simulink model "VirtualVehicleTemplate"  (R2024a)
settings: configuration reference "VehicleVariable" (kept outside this file)
StartFcn:
  | %tic
StopFcn:
  | %toc
model workspace (MAT data in the model file):
  ExtDrvCmdsSwitch : Simulink.Parameter (value not decoded)
  ExtDrvRefSwitch : Simulink.Parameter (value not decoded)
  ExtEnvSwitch : Simulink.Parameter (value not decoded)
  ExtGndSwitch : Simulink.Parameter (value not decoded)
symbols that are objects in the model workspace (value not decoded): ExtDrvCmdsSwitch, ExtDrvRefSwitch, ExtEnvSwitch, ExtGndSwitch
undefined symbols (not defined in the file): AccelCmd, AmbTemp, BaroPress, CurvGradRef, CurvRef, DCM, DecelCmd, Disabled, DriverAeroRes, DriverDrivelineRes, DriverInitialGear, DriverPreviewDist, DriverRollRes, DriverShiftTime, DriverTimeConst, DriverTractiveForce, EnvAbsPrs, EnvAirTemp, EnvGrvty, EnvNomFrictionScaling, EnvNominalGrade, EnvWindVelX, EnvWindVelY, EnvWindVelZ, FTP75, Gnd, Grade, HazzardCmd, HighBeamCmd, lambda_mux, LeftSignalCmd, LngRef, LowBeamCmd, LtrRef, PhiRef, PlntVehDstCGFrntAxl, PlntVehDstCGRearAxl, PlntVehInitLatPos, PlntVehInitLongPos, PlntVehInitPitchAng, PlntVehInitRollAng, PlntVehInitVertPos, PlntVehInitYawAng, PlntVehMass, PlntVehTrckWdth, PlntVehYawMomentInertia, PlntWhlLdRadius, RightSignalCmd, ScnCRMaxLatAccel, ScnCRRadius, ScnDLCGateLongPos, ScnDLCLatRef, ScnDLCLatRefOffset, ScnDLCLongRefBpt, ScnDLCLongRefStartPos, ScnDLCVehicleWidth, ScnFHCounterDwellTime, ScnFHInitialDwellTime, ScnFHReturnTime, ScnFHRollRateZeroCross ... (+20)
libraries: simulink x27, autolibutils x8, vehdynlibscenariocommon x7, vehdynlibviscommon x4, autolibshared x3, vehdynlibdriver x2, sim3dgroundtruthsensorlib x2, sim3dautolib x2, vrlib x1, autolibsharedcommon x1, sharedtransform x1, sim3dlib x1
(part 2 of 6)

== system VirtualVehicleTemplate/Controllers/TCU Input ==
  CntrlRx : Inport
  Brake : Inport  Port=2
  Bus Selector : BusSelector  OutputSignals=ABSFlag
  Bus Selector1 : BusSelector  OutputSignals=Driver.AccelFdbk,Driver.DecelFdbk,Driver.GearFdbk,Trans.Info.Eng.EngSpd,FrntWheels.Wheels.Omega,RearWheels.Wheels.Omega,Body.BdyFrm.Cg.Vel.xdot
  Bus to Vector : BusToVector
  Bus to Vector1 : BusToVector
  Ground : Ground
  Ground1 : Ground
  Rate Transition{1..8,23} (9 alike) : RateTransition  Deterministic=off
  Vector Concatenate : Concatenate
  <AccFdbk> : Outport
  <DecelFdbk> : Outport  Port=2
  <GearFdbk> : Outport  Port=3
  <EngSpd> : Outport  Port=4
  <Omega> : Outport  Port=5
  <Vehicle> : Outport  Port=6
  ABSFlag : Outport  Port=7
  UpReq : Outport  Port=8
  DnReq : Outport  Port=9
  wires:
  Bus Selector1/7 -> Rate Transition5/1  "<xdot>"
  Bus Selector1/2 -> Rate Transition1/1  "<DecelFdbk>"
  Ground/1 -> Rate Transition7/1
  CntrlRx/1 -> Bus Selector1/1
  Bus Selector1/1 -> Rate Transition23/1  "<AccelFdbk>"
  Vector Concatenate/1 -> Rate Transition4/1
  Bus Selector1/4 -> Rate Transition3/1  "<EngSpd>"
  Bus Selector1/3 -> Rate Transition2/1  "<GearFdbk>"
  Ground1/1 -> Rate Transition8/1
  Bus Selector/1 -> Rate Transition6/1  "<ABSFlag>"
  Brake/1 -> Bus Selector/1
  Rate Transition23/1 -> <AccFdbk>/1
  Rate Transition1/1 -> <DecelFdbk>/1
  Rate Transition2/1 -> <GearFdbk>/1
  Rate Transition3/1 -> <EngSpd>/1
  Rate Transition4/1 -> <Omega>/1
  Rate Transition5/1 -> <Vehicle>/1
  Rate Transition6/1 -> ABSFlag/1
  Rate Transition7/1 -> UpReq/1
  Rate Transition8/1 -> DnReq/1
  Bus Selector1/5 -> Bus to Vector/1  "<Omega>"
  Bus Selector1/6 -> Bus to Vector1/1  "<Omega>"
  Bus to Vector/1 -> Vector Concatenate/1
  Bus to Vector1/1 -> Vector Concatenate/2

== system VirtualVehicleTemplate/Controllers/TCU Output ==
  GearCmd : Inport
  Bus Creator1 : BusCreator  Inputs=1
  First Order Hold : FirstOrderHold  ErrorTolerance=inf
  Trans : Outport
  wires:
  Bus Creator1/1 -> Trans/1  "Trans"
  GearCmd/1 -> First Order Hold/1  "GearCmd"
  First Order Hold/1 -> Bus Creator1/1  "GearCmd"

== system VirtualVehicleTemplate/Controllers/Thermal Input ==
  Bus Element In : Inport  PortName=CntrlRx  Element=Thermal.BattCoolTemp
  Bus Element In2 : Inport  PortName=CntrlRx  Element=Thermal.CondPress
  Bus Element In3 : Inport  PortName=CntrlRx  Element=Thermal.ChlrPress
  Bus Element In5 : Inport  PortName=CntrlRx  Element=Thermal.MotorTemp
  Bus Element In6 : Inport  PortName=CntrlRx  Element=Thermal.BattTemp
  Bus Element In7 : Inport  PortName=CntrlRx  Element=Thermal.InvCoolTempOut
  Bus Element In8 : Inport  PortName=CntrlRx  Element=Thermal.InvTemp
  Bus Element In1 : Inport  PortName=CntrlRx  Element=Battery.BMSSensors.CellTemperatures
  Bus Element In4 : Inport  PortName=CntrlRx  Element=Env.AmbTemp
  Rate Transition{,1..8} (9 alike) : RateTransition
  CoolTemp : Outport
  CellTemps : Outport  Port=2
  AmbTemp : Outport  Port=3
  CondPress : Outport  Port=4
  ChlrPress : Outport  Port=5
  MotorTemp : Outport  Port=6
  BattTemp : Outport  Port=7
  InvCoolTempOut : Outport  Port=8
  InvTemp : Outport  Port=9
  wires:
  Bus Element In/1 -> Rate Transition/1
  Bus Element In1/1 -> Rate Transition8/1
  Rate Transition/1 -> CoolTemp/1
  Bus Element In2/1 -> Rate Transition1/1
  Rate Transition1/1 -> CondPress/1
  Rate Transition2/1 -> ChlrPress/1
  Bus Element In3/1 -> Rate Transition2/1
  Rate Transition3/1 -> AmbTemp/1
  Bus Element In4/1 -> Rate Transition3/1
  Rate Transition4/1 -> MotorTemp/1
  Bus Element In5/1 -> Rate Transition4/1
  Rate Transition5/1 -> BattTemp/1
  Bus Element In6/1 -> Rate Transition5/1
  Rate Transition6/1 -> InvCoolTempOut/1
  Bus Element In7/1 -> Rate Transition6/1
  Rate Transition7/1 -> InvTemp/1
  Bus Element In8/1 -> Rate Transition7/1
  Rate Transition8/1 -> CellTemps/1

== system VirtualVehicleTemplate/Controllers/Thermal Management ==
  CoolTemp : Inport
  CellTemps : Inport  Port=2
  AmbTemp : Inport  Port=3  Unit=K
  CondPress : Inport  Port=4
  ChlrPress : Inport  Port=5
  MotorTemp : Inport  Port=6
  BattTemp : Inport  Port=7
  InvCoolTempOut : Inport  Port=8
  InvTemp : Inport  Port=9
  NoThermalControl : ModelReference  ModelNameDialog=NoThermalControl  SimulationMode=Normal  VariantControl=NoThermalControl  ModelReferenceVersion=2.28
  ThermalControl : ModelReference  ModelNameDialog=ThermalControl.slx  SimulationMode=Normal  VariantControl=ThermalControl  ModelReferenceVersion=2.119
  ThermalControlGen1 : ModelReference  ModelNameDialog=ThermalControlGen1  SimulationMode=Normal  VariantControl=ThermalControlGen1  ModelReferenceVersion=2.30
  ValveCmd : Outport
  PumpCmd : Outport  Port=2
  CmpCmd : Outport  Port=3
  FanCmd : Outport  Port=4
  HeaterCmd : Outport  Port=5
  MotPmpCmd : Outport  Port=6
  BattPmpCmd : Outport  Port=7
  ChlrByPCmd : Outport  Port=8
  SerParCmd : Outport  Port=9
  RadByPCmd : Outport  Port=10

== system VirtualVehicleTemplate/Controllers/Thermal Output ==
  ValveCmd : Inport
  PumpCmd : Inport  Port=2
  CmpCmd : Inport  Port=3
  FanCmd : Inport  Port=4
  HeaterCmd : Inport  Port=5
  MotPmpCmd : Inport  Port=6
  BattPmpCmd : Inport  Port=7
  ChlrPyPCmd : Inport  Port=8
  SerParCmd : Inport  Port=9
  RadByPCmd : Inport  Port=10
  First Order Hold{,1..9} (10 alike) : FirstOrderHold  ErrorTolerance=inf
  Bus Element Out : Outport  PortName=Thermal  Element=ValveCmd
  Bus Element Out1 : Outport  PortName=Thermal  Element=PumpCmd
  Bus Element Out2 : Outport  PortName=Thermal  Element=CmpCmd
  Bus Element Out3 : Outport  PortName=Thermal  Element=FanCmd
  Bus Element Out4 : Outport  PortName=Thermal  Element=HeaterCmd
  Bus Element Out5 : Outport  PortName=Thermal  Element=MotPmpCmd
  Bus Element Out6 : Outport  PortName=Thermal  Element=BattPmpCmd
  Bus Element Out7 : Outport  PortName=Thermal  Element=ChlrByPCmd
  Bus Element Out8 : Outport  PortName=Thermal  Element=SerParCmd
  Bus Element Out9 : Outport  PortName=Thermal  Element=RadByPCmd
  wires:
  PumpCmd/1 -> First Order Hold1/1
  ValveCmd/1 -> First Order Hold/1
  First Order Hold/1 -> Bus Element Out/1
  First Order Hold1/1 -> Bus Element Out1/1
  CmpCmd/1 -> First Order Hold2/1
  First Order Hold2/1 -> Bus Element Out2/1
  First Order Hold3/1 -> Bus Element Out3/1
  FanCmd/1 -> First Order Hold3/1
  HeaterCmd/1 -> First Order Hold4/1
  First Order Hold4/1 -> Bus Element Out4/1
  MotPmpCmd/1 -> First Order Hold5/1
  First Order Hold5/1 -> Bus Element Out5/1
  BattPmpCmd/1 -> First Order Hold6/1
  First Order Hold6/1 -> Bus Element Out6/1
  ChlrPyPCmd/1 -> First Order Hold7/1
  First Order Hold7/1 -> Bus Element Out7/1
  First Order Hold8/1 -> Bus Element Out8/1
  SerParCmd/1 -> First Order Hold8/1
  First Order Hold9/1 -> Bus Element Out9/1
  RadByPCmd/1 -> First Order Hold9/1

== system VirtualVehicleTemplate/Controllers/Transmission Control Unit (TCU) ==
  Accel : Inport
  BrkCmd : Inport  Port=2
  GearReq : Inport  Port=3
  EngSpd : Inport  Port=4
  Omega : Inport  Port=5  Unit=rad/s
  VehSpdFdbk : Inport  Port=6
  ABSFlag : Inport  Port=7
  UpReq : Inport  Port=8
  DownReq : Inport  Port=9  Unit=rad/s
  DriverPassThrough : ModelReference  ModelNameDialog=DriverPassThrough.slx  VariantControl=DriverPassThrough  ModelReferenceVersion=8.0
  TransmissionController : ModelReference  ModelNameDialog=TransmissionController  VariantControl=TransmissionController  ModelReferenceVersion=8.8
  " Gear" : Outport  VectorParamsAs1DForOutWhenUnconnected=off

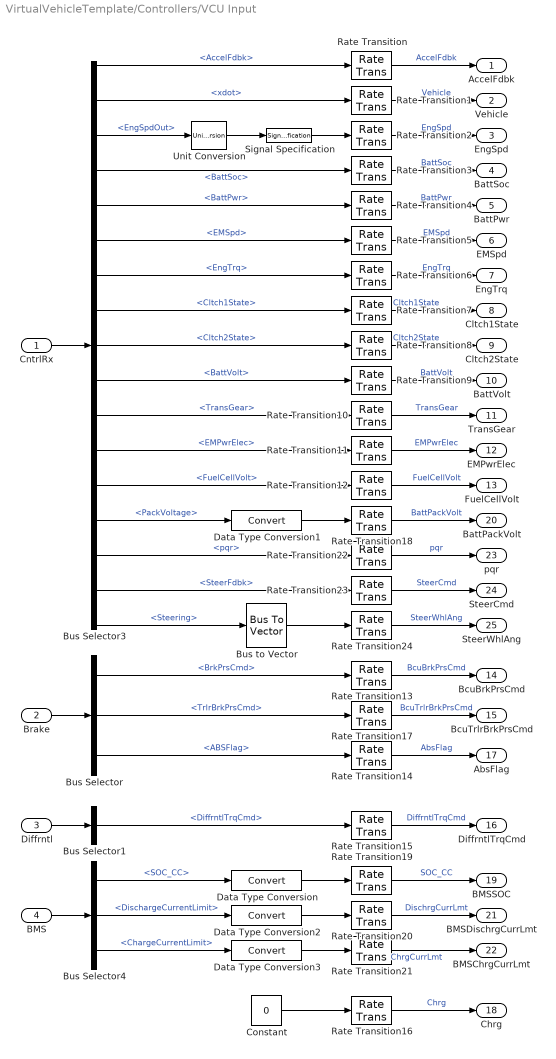
== system VirtualVehicleTemplate/Controllers/VCU Input ==
  CntrlRx : Inport
  Brake : Inport  Port=2
  Diffrntl : Inport  Port=3
  BMS : Inport  Port=4
  Bus Selector : BusSelector  OutputSignals=BrkPrsCmd,TrlrBrkPrsCmd,ABSFlag
  Bus Selector1 : BusSelector  OutputSignals=DiffrntlTrqCmd
  Bus Selector3 : BusSelector  OutputSignals=Driver.AccelFdbk,Body.BdyFrm.Cg.Vel.xdot,Engine.EngSpdOut,Battery.BattInfo.BattSoc,Battery.BattInfo.BattPwr,EM.EMSpd,Engine.EngTrq,Trans.Cltch1State,Trans.Cltch2State,Battery.BattInfo.BattVolt,Trans.Info.Trans.TransGear,EM.EMPwrElec,FuelCell.FuelCellVolt,Battery.BMSSensors.PackVoltage,IMU.pqr,Driver.SteerFdbk,Steering
  Bus Selector4 : BusSelector  OutputSignals=BMSInfo.SOC.SOC_CC,BMSCmd.CurrentLimitsBus.DischargeCurrentLimit,BMSCmd.CurrentLimitsBus.ChargeCurrentLimit
  Bus to Vector : BusToVector
  Constant : Constant  Value=0  SampleTime=-1
  Data Type Conversion{,1..3} (4 alike) : DataTypeConversion  SaturateOnIntegerOverflow=off  RndMeth=Floor
  Rate Transition{,1..24} (25 alike) : RateTransition  Deterministic=off
  Signal Specification : SignalSpecification  Unit=rad/s
  Unit Conversion : UnitConversion
  AccelFdbk : Outport
  Vehicle : Outport  Port=2
  EngSpd : Outport  Port=3
  BattSoc : Outport  Port=4
  BattPwr : Outport  Port=5
  EMSpd : Outport  Port=6
  EngTrq : Outport  Port=7
  Cltch1State : Outport  Port=8
  Cltch2State : Outport  Port=9
  BattVolt : Outport  Port=10
  TransGear : Outport  Port=11
  EMPwrElec : Outport  Port=12
  FuelCellVolt : Outport  Port=13
  BcuBrkPrsCmd : Outport  Port=14
  BcuTrlrBrkPrsCmd : Outport  Port=15
  DiffrntlTrqCmd : Outport  Port=16
  AbsFlag : Outport  Port=17
  Chrg : Outport  Port=18
  BMSSOC : Outport  Port=19
  BattPackVolt : Outport  Port=20
  BMSDischrgCurrLmt : Outport  Port=21
  BMSChrgCurrLmt : Outport  Port=22
  pqr : Outport  Port=23
  SteerCmd : Outport  Port=24
  SteerWhlAng : Outport  Port=25
  wires:
  Bus Selector3/5 -> Rate Transition4/1  "<BattPwr>"
  Bus Selector3/1 -> Rate Transition/1  "<AccelFdbk>"
  Bus Selector3/7 -> Rate Transition6/1  "<EngTrq>"
  Bus Selector3/4 -> Rate Transition3/1  "<BattSoc>"
  Bus Selector3/6 -> Rate Transition5/1  "<EMSpd>"
  CntrlRx/1 -> Bus Selector3/1
  Bus Selector3/11 -> Rate Transition10/1  "<TransGear>"
  Bus Selector3/9 -> Rate Transition8/1  "<Cltch2State>"
  Bus Selector3/13 -> Rate Transition12/1  "<FuelCellVolt>"
  Bus Selector3/2 -> Rate Transition1/1  "<xdot>"
  Bus Selector3/8 -> Rate Transition7/1  "<Cltch1State>"
  Bus Selector3/10 -> Rate Transition9/1  "<BattVolt>"
  Bus Selector3/3 -> Unit Conversion/1  "<EngSpdOut>"
  Bus Selector3/12 -> Rate Transition11/1  "<EMPwrElec>"
  Bus Selector/1 -> Rate Transition13/1  "<BrkPrsCmd>"
  Constant/1 -> Rate Transition16/1
  Brake/1 -> Bus Selector/1
  Bus Selector/3 -> Rate Transition14/1  "<ABSFlag>"
  Diffrntl/1 -> Bus Selector1/1
  Bus Selector1/1 -> Rate Transition15/1  "<DiffrntlTrqCmd>"
  Rate Transition/1 -> AccelFdbk/1  "AccelFdbk"
  Rate Transition1/1 -> Vehicle/1  "Vehicle"
  Rate Transition2/1 -> EngSpd/1  "EngSpd"
  Rate Transition3/1 -> BattSoc/1  "BattSoc"
  Rate Transition4/1 -> BattPwr/1  "BattPwr"
  Rate Transition5/1 -> EMSpd/1  "EMSpd"
  Rate Transition6/1 -> EngTrq/1  "EngTrq"
  Rate Transition7/1 -> Cltch1State/1  "Cltch1State"
  Rate Transition8/1 -> Cltch2State/1  "Cltch2State"
  Rate Transition9/1 -> BattVolt/1  "BattVolt"
  Rate Transition10/1 -> TransGear/1  "TransGear"
  Rate Transition11/1 -> EMPwrElec/1  "EMPwrElec"
  Rate Transition12/1 -> FuelCellVolt/1  "FuelCellVolt"
  Rate Transition13/1 -> BcuBrkPrsCmd/1  "BcuBrkPrsCmd"
  Rate Transition14/1 -> AbsFlag/1  "AbsFlag"
  Rate Transition15/1 -> DiffrntlTrqCmd/1  "DiffrntlTrqCmd"
  Rate Transition16/1 -> Chrg/1  "Chrg"
  Rate Transition20/1 -> BMSDischrgCurrLmt/1  "DischrgCurrLmt"
  Rate Transition19/1 -> BMSSOC/1  "SOC_CC"
  Rate Transition21/1 -> BMSChrgCurrLmt/1  "ChrgCurrLmt"
  Data Type Conversion3/1 -> Rate Transition21/1
  Data Type Conversion2/1 -> Rate Transition20/1
  Bus Selector4/1 -> Data Type Conversion/1  "<SOC_CC>"
  Data Type Conversion/1 -> Rate Transition19/1
  Bus Selector4/3 -> Data Type Conversion3/1  "<ChargeCurrentLimit>"
  Bus Selector4/2 -> Data Type Conversion2/1  "<DischargeCurrentLimit>"
  BMS/1 -> Bus Selector4/1
  Data Type Conversion1/1 -> Rate Transition18/1
  Rate Transition18/1 -> BattPackVolt/1  "BattPackVolt"
  Bus Selector3/14 -> Data Type Conversion1/1  "<PackVoltage>"
  Bus Selector/2 -> Rate Transition17/1  "<TrlrBrkPrsCmd>"
  Rate Transition17/1 -> BcuTrlrBrkPrsCmd/1  "BcuTrlrBrkPrsCmd"
  Rate Transition22/1 -> pqr/1  "pqr"
  Rate Transition23/1 -> SteerCmd/1  "SteerCmd"
  Rate Transition24/1 -> SteerWhlAng/1  "SteerWhlAng"
  Bus Selector3/15 -> Rate Transition22/1  "<pqr>"
  Bus Selector3/16 -> Rate Transition23/1  "<SteerFdbk>"
  Bus Selector3/17 -> Bus to Vector/1  "<Steering>"
  Unit Conversion/1 -> Signal Specification/1
  Signal Specification/1 -> Rate Transition2/1
  Bus to Vector/1 -> Rate Transition24/1

== system VirtualVehicleTemplate/Controllers/VCU Output ==
  EngTrqCmd : Inport
  EMTrqCmd : Inport  Port=2
  VcuBrkPrsCmd : Inport  Port=3
  VcuTrlrBrkPrsCmd : Inport  Port=4
  Cltch1Cmd : Inport  Port=5
  Neutral : Inport  Port=6
  FuelCellCurrCmd : Inport  Port=7
  FuelCellTempCmd : Inport  Port=8
  First Order Hold{,1..2,4..7} (7 alike) : FirstOrderHold  ErrorTolerance=inf
  First Order Hold3 : FirstOrderHold  ErrorTolerance=inf  AllowContinuousInput=on
  Out Bus Element : Outport  PortName=Vcu  Element=EngTrqCmd
  Out Bus Element1 : Outport  PortName=Vcu  Element=EMTrqCmd
  Out Bus Element2 : Outport  PortName=Vcu  Element=VcuBrkPrsCmd
  Out Bus Element3 : Outport  PortName=Vcu  Element=VcuTrlrBrkPrsCmd
  Out Bus Element4 : Outport  PortName=Vcu  Element=Cltch1Cmd
  Out Bus Element5 : Outport  PortName=Vcu  Element=Neutral
  Out Bus Element6 : Outport  PortName=Vcu  Element=FuelCellCurrCmd
  Out Bus Element7 : Outport  PortName=Vcu  Element=FuelCellTempCmd
  Out Bus Element8 : Outport  Port=2  PortName=VcuFdbk  Element=EngTrqCmd
  Out Bus Element9 : Outport  Port=2  PortName=VcuFdbk  Element=EMTrqCmd
  Out Bus Element10 : Outport  Port=2  PortName=VcuFdbk  Element=VcuBrkPrsCmd
  Out Bus Element11 : Outport  Port=2  PortName=VcuFdbk  Element=VcuTrlrBrkPrsCmd
  Out Bus Element12 : Outport  Port=2  PortName=VcuFdbk  Element=Cltch1Cmd
  Out Bus Element13 : Outport  Port=2  PortName=VcuFdbk  Element=Neutral
  Out Bus Element14 : Outport  Port=2  PortName=VcuFdbk  Element=FuelCellCurrCmd
  Out Bus Element15 : Outport  Port=2  PortName=VcuFdbk  Element=FuelCellTempCmd
  wires:
  Cltch1Cmd/1 -> Out Bus Element12/1, First Order Hold4/1  "Cltch1Cmd"
  EngTrqCmd/1 -> Out Bus Element8/1, First Order Hold/1  "EngTrqCmd"
  VcuBrkPrsCmd/1 -> Out Bus Element10/1, First Order Hold2/1  "VcuBrkPrsCmd"
  Neutral/1 -> Out Bus Element13/1, First Order Hold5/1  "Neutral"
  FuelCellCurrCmd/1 -> Out Bus Element14/1, First Order Hold6/1  "FuelCellCurrCmd"
  EMTrqCmd/1 -> Out Bus Element9/1, First Order Hold1/1  "EMTrqCmd"
  FuelCellTempCmd/1 -> Out Bus Element15/1, First Order Hold7/1  "FuelCellTempCmd"
  VcuTrlrBrkPrsCmd/1 -> Out Bus Element11/1, First Order Hold3/1  "VcuTrlrBrkPrsCmd"
  First Order Hold/1 -> Out Bus Element/1
  First Order Hold1/1 -> Out Bus Element1/1
  First Order Hold2/1 -> Out Bus Element2/1
  First Order Hold3/1 -> Out Bus Element3/1
  First Order Hold4/1 -> Out Bus Element4/1
  First Order Hold5/1 -> Out Bus Element5/1
  First Order Hold6/1 -> Out Bus Element6/1
  First Order Hold7/1 -> Out Bus Element7/1

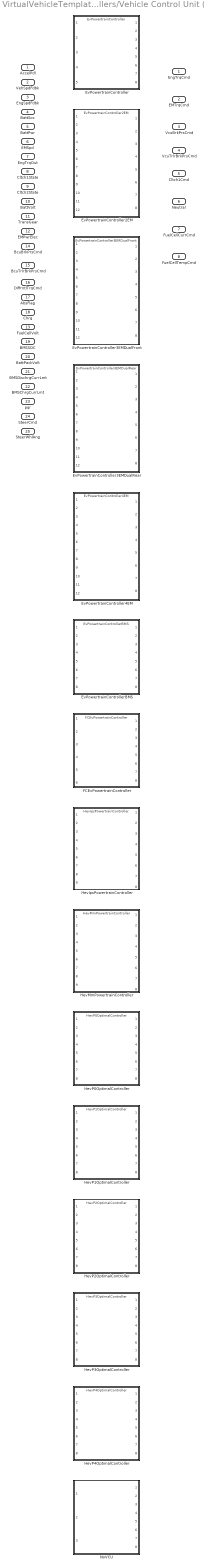
== system VirtualVehicleTemplate/Controllers/Vehicle Control Unit (VCU) ==
  AccelPdl : Inport
  VehSpdFdbk : Inport  Port=2
  EngSpdFdbk : Inport  Port=3
  BattSoc : Inport  Port=4
  BattPwr : Inport  Port=5
  EMSpd : Inport  Port=6
  EngTrqOut : Inport  Port=7
  Cltch1State : Inport  Port=8
  Cltch2State : Inport  Port=9
  BattVolt : Inport  Port=10
  TransGear : Inport  Port=11
  EMPwrElec : Inport  Port=12
  FuelCellVolt : Inport  Port=13
  BcuBrkPrsCmd : Inport  Port=14
  BcuTrlrBrkPrsCmd : Inport  Port=15
  DiffrntlTrqCmd : Inport  Port=16
  AbsFlag : Inport  Port=17
  Chrg : Inport  Port=18
  BMSSOC : Inport  Port=19
  BattPackVolt : Inport  Port=20
  BMSDischrgCurrLmt : Inport  Port=21
  BMSChrgCurrLmt : Inport  Port=22
  pqr : Inport  Port=23
  SteerCmd : Inport  Port=24
  SteerWhlAng : Inport  Port=25
  EvPowertrainController : ModelReference  ModelNameDialog=EvPowertrainController  VariantControl=EvPowertrainController  ModelReferenceVersion=8.2
  EvPowertrainController2EM : ModelReference  ModelNameDialog=EvPowertrainController2EM.slx  VariantControl=EvPowertrainController2EM  ModelReferenceVersion=8.3
  EvPowertrainController3EMDualFront : ModelReference  ModelNameDialog=EvPowertrainController3EMDualFront.slx  VariantControl=EvPowertrainController3EMDualFront  ModelReferenceVersion=8.3
  EvPowertrainController3EMDualRear : ModelReference  ModelNameDialog=EvPowertrainController3EMDualRear.slx  VariantControl=EvPowertrainController3EMDualRear  ModelReferenceVersion=8.3
  EvPowertrainController4EM : ModelReference  ModelNameDialog=EvPowertrainController4EM.slx  VariantControl=EvPowertrainController4EM  ModelReferenceVersion=8.3
  EvPowertrainControllerBMS : ModelReference  ModelNameDialog=EvPowertrainControllerBMS.slx  VariantControl=EvPowertrainControllerBMS  ModelReferenceVersion=8.2
  FCEvPowertrainController : ModelReference  ModelNameDialog=FCEvPowertrainController  VariantControl=FCEvPowertrainController  ModelReferenceVersion=8.1
  HevIpsPowertrainController : ModelReference  ModelNameDialog=HevIpsPowertrainController  VariantControl=HevIpsPowertrainController  ModelReferenceVersion=13.7
  HevMmPowertrainController : ModelReference  ModelNameDialog=HevMmPowertrainController  VariantControl=HevMmPowertrainController  ModelReferenceVersion=13.1
  HevP0OptimalController : ModelReference  ModelNameDialog=HevP0OptimalController  VariantControl=HevP0OptimalController  ModelReferenceVersion=8.4
  HevP1OptimalController : ModelReference  ModelNameDialog=HevP1OptimalController  VariantControl=HevP1OptimalController  ModelReferenceVersion=8.4
  HevP2OptimalController : ModelReference  ModelNameDialog=HevP2OptimalController  VariantControl=HevP2OptimalController  ModelReferenceVersion=8.4
  HevP3OptimalController : ModelReference  ModelNameDialog=HevP3OptimalController  VariantControl=HevP3OptimalController  ModelReferenceVersion=8.4
  HevP4OptimalController : ModelReference  ModelNameDialog=HevP4OptimalController  VariantControl=HevP4OptimalController  ModelReferenceVersion=8.4
  NoVCU : Subsystem  VariantControl=NoVCU  ReferencedSubsystem=NoVCU
  EngTrqCmd : Outport  VectorParamsAs1DForOutWhenUnconnected=off
  EMTrqCmd : Outport  Port=2  VectorParamsAs1DForOutWhenUnconnected=off
  VcuBrkPrsCmd : Outport  Port=3  VectorParamsAs1DForOutWhenUnconnected=off
  VcuTrlrBrkPrsCmd : Outport  Port=4  VectorParamsAs1DForOutWhenUnconnected=off
  Cltch1Cmd : Outport  Port=5  VectorParamsAs1DForOutWhenUnconnected=off
  Neutral : Outport  Port=6  VectorParamsAs1DForOutWhenUnconnected=off
  FuelCellCurrCmd : Outport  Port=7  VectorParamsAs1DForOutWhenUnconnected=off
  FuelCellTempCmd : Outport  Port=8  VectorParamsAs1DForOutWhenUnconnected=off

== system VirtualVehicleTemplate/Driver Commands/Driver Commands ==
  VehRef : Inport
  VehFdbk : Inport  Port=2
  Env : Inport  Port=3
  SteerCmd : Inport  Port=4
  AccelCmd : Inport  Port=5
  BrakeCmd : Inport  Port=6
  GearCmd : Inport  Port=7
  Dashboard Widgets : Subsystem  VariantControl=driverType==5
  Game Wheel Hardware : Subsystem  VariantControl=driverType==6
  Longitudinal Driver : Subsystem  VariantControl=driverType==1
  No Driver : Subsystem  VariantControl=driverType==7
  Open Loop : Subsystem  VariantControl=driverType==4
  Predictive Driver : Subsystem  VariantControl=driverType==2
  Predictive Stanley Driver : Subsystem  VariantControl=driverType==3
  " Driver" : Outport  VectorParamsAs1DForOutWhenUnconnected=off

== system VirtualVehicleTemplate/Environment/Ground Feedback ==
  Friction : Inport
  WheelFdbk : Inport  Port=2
  3D Engine : Subsystem  VariantControl=1
  Constant : Subsystem  VariantControl=0
  Three-Axle Constant : Subsystem  VariantControl=2
  Gnd : Outport  VectorParamsAs1DForOutWhenUnconnected=off

== system VirtualVehicleTemplate/Environment/Subsystem ==
  ExtEnv : Inport
  ExtGnd : Inport  Port=2
  AmbTemp : Inport  Port=3
  BaroPress : Inport  Port=4
  Wind : Inport  Port=5
  InGnd : Inport  Port=6
  Bus Assignment : BusAssignment  AssignedSignals=AmbTemp,BaroPress,Wind,Grade
  Bus Assignment1 : BusAssignment  AssignedSignals=Z,DCM,lambda_mux
  Bus Assignment2 : BusAssignment  AssignedSignals=BaroPress,AmbTemp,Wind,Grade,Gnd
  Bus Selector : BusSelector  OutputSignals=BaroPress,AmbTemp,Wind,Grade
  Estimated Grade : Subsystem
  ExtEnvSwitch : Constant  Value=ExtEnvSwitch  SampleTime=-1
  ExtGndSwitch : Constant  Value=ExtGndSwitch  SampleTime=-1
  Switch : Switch  Criteria=u2 > Threshold  SaturateOnIntegerOverflow=off  InputSameDT=off
  Switch1 : Switch  Criteria=u2 > Threshold  SaturateOnIntegerOverflow=off  InputSameDT=off
  To Virtual Bus : SignalConversion  ConversionOutput=Virtual bus  OverrideOpt=off
  VVCEnv : Constant  Value=0  OutDataTypeStr=Bus: VVCEnvGndBUS  SampleTime=-1
  Variant Subsystem : Subsystem  Variant=on  VariantControlMode=label  LabelModeActiveChoice=TwoAxle
  Env : Outport
  wires:
  Bus Assignment1/1 -> Switch1/3
  Estimated Grade/1(Grade) -> Bus Assignment/5
  ExtGndSwitch/1 -> Switch1/2
  ExtEnv/1 -> Switch/1, Bus Assignment/1
  InGnd/1 -> Variant Subsystem/1(InGnd), Estimated Grade/1(Gnd)
  ExtEnvSwitch/1 -> Switch/2
  Bus Assignment/1 -> Switch/3
  BaroPress/1 -> Bus Assignment/3
  VVCEnv/1 -> Bus Assignment2/1
  Switch1/1 -> Bus Assignment2/6
  ExtGnd/1 -> Switch1/1, Bus Assignment1/1
  Wind/1 -> Bus Assignment/4
  Bus Selector/1 -> Bus Assignment2/2  "<BaroPress>"
  Switch/1 -> Bus Selector/1
  Bus Selector/2 -> Bus Assignment2/3  "<AmbTemp>"
  Bus Assignment2/1 -> To Virtual Bus/1
  Bus Selector/4 -> Bus Assignment2/5  "<Grade>"
  Bus Selector/3 -> Bus Assignment2/4  "<Wind>"
  AmbTemp/1 -> Bus Assignment/2
  To Virtual Bus/1 -> Env/1
  Variant Subsystem/1(z) -> Bus Assignment1/2
  Variant Subsystem/2(<DCM>) -> Bus Assignment1/3
  Variant Subsystem/3(lambda_mux) -> Bus Assignment1/4

== system VirtualVehicleTemplate/Environment/Varying Friction ==
  In1 : Inport
  In2 : Inport  Port=2
  Cg : Inport  Port=3
  Constant Friction : Subsystem  VariantControl=0
  Three-Axle Constant Friction : Subsystem  VariantControl=2
  Varying Friction : Subsystem  VariantControl=1
  FricCoeffLambda : Outport

== system VirtualVehicleTemplate/Scenarios/Coordinate Systems ==
  ExtDrvRefIn : Inport
  ExtDrvCmdIn : Inport  Port=2
  ISO 8855 (Z-up) : Subsystem  VariantControl=Choice
  SAE J670 (Z-down) : Subsystem  VariantControl=ISO 8855 (Z-up)1
  ExtDrvRef : Outport
  ExtDrvCmd : Outport  Port=2

== system VirtualVehicleTemplate/Scenarios/Reference Generator ==
  note: 1) Add Subsystem or Model blocks as valid variant choices.
      | 2) You cannot connect blocks at this level. At simulation, connectivity is automatically
      | determined, based on the active variant and port name matching.
  VehFdbk : Inport
  Drive Cycle : Subsystem  VariantControl=Drive Cycle
  Reference Generator : Subsystem  Priority=1  VariantControl=Vehicle Dynamic Scenarios  mask(Reference Generator){manType=Drive Cycle, manOverride=off, prevType=Drive Cycle, t_start=ScnStartTime, xdot_r=ScnLongVelRef, xdotUnit=mph, steerDir=off, aMode=2, omega_hw=ScnISHandwheelRate, theta_max=ScnISMaxHandwheelAng, t_stop=ScnISSteerHoldTime, ay_max=ScnISMaxLatAccel, ay_stop=off, XGate=ScnDLCGateLongPos, xStart=ScnDLCLongRefStartPos, vehW=ScnDLCVehicleWidth, latoff=ScnDLCLatRefOffset, latRefbp=ScnDLCLongRefBpt, latRef=ScnDLCLatRef, t_sweep=ScnSSSweepTime, theta_hw=ScnSSSteerAmp, theta_hw_final=ScnSSFinalFreq, steerF=ScnSDSteerFreq, steerA=ScnSDSteerAmp, tdwell=ScnSDDwellTime, R=ScnCRRadius, cr_ay_max=ScnCRMaxLatAccel, cr_ay_stop=off, steerRate=ScnFHSteerSpeed, steerAFH=ScnFHSteerAmp, pFdbk=off, tDwell1=ScnFHInitialDwellTime, tDwell2=ScnFHCounterDwellTime, tSteer3=ScnFHReturnTime, pZero=ScnFHRollRateZeroCross, cycleVar=FTP75, ax=.5, ax_dec=.5, fixhw=on, x_brake=175, t_wot2=ScnTimeToStrtDecel, simTime=2474, engine3D=Disabled, Trailer=No Trailer, SceneDesc=Open surface, dt3D=.03, defaultPos=User-specified, X_o=PlntVehInitLongPos, Y_o=PlntVehInitLatPos, Z_o=PlntVehInitVertPos, phi_o=PlntVehInitRollAng, theta_o=PlntVehInitPitchAng, psi_o=PlntVehInitYawAng}
      mask prompts: manType "vdynblks:vehdynManConstantRadius:blkPrm_manType"; manOverride "vdynblks:vehdynManConstantRadius:blkPrm_manOverride"; t_start "vdynblks:vehdynManConstantRadius:blkPrm_t_start"; xdot_r "vdynblks:vehdynManConstantRadius:blkPrm_xdot_r"; xdotUnit "vdynblks:vehdynManStraightBrake:blkPrm_xdotUnit"; steerDir "Change direction, steerDir"; omega_hw "vdynblks:vehdynManConstantRadius:blkPrm_omega_hw"; theta_max "vdynblks:vehdynManConstantRadius:blkPrm_theta_max"; t_stop "vdynblks:vehdynManConstantRadius:blkPrm_t_stop"; ay_max "vdynblks:vehdynManConstantRadius:blkPrm_ay_max"; ay_stop "vdynblks:vehdynManConstantRadius:blkPrm_ay_stop"; XGate "vdynblks:vehdynManConstantRadius:blkPrm_XGate"; xStart "vdynblks:vehdynManConstantRadius:blkPrm_xStart"; vehW "vdynblks:vehdynManConstantRadius:blkPrm_vehW"; latoff "vdynblks:vehdynManConstantRadius:blkPrm_latoff"; latRefbp "vdynblks:vehdynManConstantRadius:blkPrm_latRefbp"; latRef "vdynblks:vehdynManConstantRadius:blkPrm_latRef"; t_sweep "vdynblks:vehdynManConstantRadius:blkPrm_t_sweep"; theta_hw "vdynblks:vehdynManConstantRadius:blkPrm_theta_hw"; theta_hw_final "vdynblks:vehdynManConstantRadius:blkPrm_theta_hw_final"; steerF "vdynblks:vehdynManConstantRadius:blkPrm_steerF"; steerA "vdynblks:vehdynManConstantRadius:blkPrm_steerA"; tdwell "vdynblks:vehdynManConstantRadius:blkPrm_tdwell"; R "Radius value, R [m]:"; cr_ay_max "Lateral acceleration absolute threshold, ay_max [g]:"; cr_ay_stop "Stop simulation at lateral acceleration threshold"; steerRate "vdynblks:vehdynManFishook:blkPrm_steerRate"; steerAFH "vdynblks:vehdynManConstantRadius:blkPrm_steerAFH"; pFdbk "vdynblks:vehdynManFishook:blkPrm_pFdbk"; tDwell1 "vdynblks:vehdynManFishook:blkPrm_tDwell1"; tDwell2 "vdynblks:vehdynManFishook:blkPrm_tDwell2"; tSteer3 "vdynblks:vehdynManFishook:blkPrm_tSteer3"; pZero "vdynblks:vehdynManFishook:blkPrm_pZero"; cycleVar "autoblks_shared:autoblkDriveCycleSource:blkPrm_cycleVar"; ax "vdynblks:vehdynManStraightBrake:blkPrm_ax"; ax_dec "vdynblks:vehdynManStraightBrake:blkPrm_ax_dec"; fixhw "vdynblks:vehdynManStraightBrake:blkPrm_fixhw"; x_brake "vdynblks:vehdynManStraightBrake:blkPrm_x_brake"; t_wot2 "autoblks_shared:autoblkDriveCycleSource:blkPrm_t_wot2"; simTime "vdynblks:vehdynManConstantRadius:blkPrm_simTime"; engine3D "vdynblks:vehdynManConstantRadius:blkPrm_engine3D"; SceneDesc "vdynblks:vehdynManConstantRadius:blkPrm_SceneDesc"; dt3D "vdynblks:vehdynManConstantRadius:blkPrm_dt3D"; X_o "Initial longitudinal position, X_o [m]:"; Y_o "Initial lateral position, Y_o [m]:"; Z_o "vdynblks:vehdynManConstantRadius:blkPrm_Z_o"; phi_o "vdynblks:vehdynManConstantRadius:blkPrm_phi_o"; theta_o "vdynblks:vehdynManConstantRadius:blkPrm_theta_o"; psi_o "Initial yaw angle, psi_o [rad]:"
      mask help: vdynblks:vehdynManConstantRadius:blkDesc
      mask init:
      | [~]=vdynblksrefconfig(gcb,0);
      settings: AttributesFormatString=%<manType>
      mask Help: eval('vdynblkshelp(''vdcrrefgen'')');
      mask TypeOptions manType: autoblks_reference:autoVirtualRefGen:blkCmb_manType_c1 | autoblks_reference:autoVirtualRefGen:blkCmb_manType_c2 | autoblks_reference:autoVirtualRefGen:blkCmb_manType_c3 | autoblks_reference:autoVirtualRefGen:blkCmb_manType_c4 | autoblks_reference:autoVirtualRefGen:blkCmb_manType_c5 | autoblks_reference:autoVirtualRefGen:blkCmb_manType_c6 | autoblks_reference:autoVirtualRefGen:blkCmb_manType_c7 | autoblks_reference:autoVirtualRefGen:blkCmb_manType_c8 | autoblks_reference:autoVirtualRefGen:blkCmb_manType_c9 | autoblks_reference:autoVirtualRefGen:blkCmb_manType_c10
      mask Callback manType:
      | [~]=vdynblksrefconfig(gcb,0);
      | [~]=vdynblksrefconfig(gcb,1);
      mask Callback manOverride: [~]=vdynblksrefconfig(gcb,3);
      mask TypeOptions prevType: autoblks_reference:autoVirtualRefGen:blkCmb_manType_c1 | autoblks_reference:autoVirtualRefGen:blkCmb_manType_c2 | autoblks_reference:autoVirtualRefGen:blkCmb_manType_c3 | autoblks_reference:autoVirtualRefGen:blkCmb_manType_c4 | autoblks_reference:autoVirtualRefGen:blkCmb_manType_c5 | autoblks_reference:autoVirtualRefGen:blkCmb_manType_c6 | autoblks_reference:autoVirtualRefGen:blkCmb_manType_c7 | autoblks_reference:autoVirtualRefGen:blkCmb_manType_c8 | autoblks_reference:autoVirtualRefGen:blkCmb_manType_c9 | autoblks_reference:autoVirtualRefGen:blkCmb_manType_c10
      mask TypeOptions xdotUnit:
      | Reference Generator/Braking/Straight Maneuver Reference
      | Generator/xdotUnit | Reference Generator/Constant Radius/Constant Radius/xdotUnit | Reference Generator/Double Lane Change/Double Lane Change/xdotUnit | Reference Generator/Drive Cycle/Drive Cycle Source/outUnit | Reference Generator/Fishhook/Fishhook/xdotUnit | Reference Generator/Increasing Steer/Increasing Steer/xdotUnit | Reference Generator/Sine with Dwell/Sine With Dwell/xdotUnit | Reference Generator/Swept Sine/Swept Sine/xdotUnit | Reference Generator/WOT/Drive Cycle Source/outUnit
      mask TypeOptions steerDir: Reference Generator/Constant Radius/Constant Radius/steerDir | Reference Generator/Fishhook/Fishhook/steerDir | Reference Generator/Increasing Steer/Increasing Steer/steerDir | Reference Generator/Sine with Dwell/Sine With Dwell/steerDir
      mask TypeOptions omega_hw: Reference Generator/Increasing Steer/Increasing Steer/omega_hw
      mask TypeOptions theta_max: Reference Generator/Increasing Steer/Increasing Steer/theta_max
      mask TypeOptions t_stop: Reference Generator/Increasing Steer/Increasing Steer/t_stop
      mask TypeOptions ay_max: Reference Generator/Increasing Steer/Increasing Steer/ay_max
      mask TypeOptions ay_stop: Reference Generator/Increasing Steer/Increasing Steer/ay_stop
      mask Callback ay_stop:
      | if strcmp(get_param(gcb,'ay_stop'),'off')
      |     autoblksenableparameters(gcb, [], {'ay_max'},[],[],true);
      | else
      |     autoblksenableparameters(gcb,{'ay_max'},[],[],[],true);
      | end
      mask TypeOptions XGate: Reference Generator/Double Lane Change/Double Lane Change/XGate
      mask TypeOptions xStart: Reference Generator/Double Lane Change/Double Lane Change/xStart
      mask TypeOptions vehW: Reference Generator/Double Lane Change/Double Lane Change/vehW
      mask TypeOptions latoff: Reference Generator/Double Lane Change/Double Lane Change/latoff
      mask TypeOptions latRefbp: Reference Generator/Double Lane Change/Double Lane Change/latRefbp
      mask TypeOptions latRef: Reference Generator/Double Lane Change/Double Lane Change/latRef
      mask TypeOptions t_sweep: Reference Generator/Swept Sine/Swept Sine/t_sweep
      mask TypeOptions theta_hw: Reference Generator/Swept Sine/Swept Sine/theta_hw
      mask TypeOptions theta_hw_final: Reference Generator/Swept Sine/Swept Sine/theta_hw_final
      mask TypeOptions steerF: Reference Generator/Sine with Dwell/Sine With Dwell/steerF
      mask TypeOptions steerA: Reference Generator/Sine with Dwell/Sine With Dwell/steerA
      mask TypeOptions tdwell: Reference Generator/Sine with Dwell/Sine With Dwell/tdwell
      mask TypeOptions R: Reference Generator/Constant Radius/Constant Radius/R
      mask TypeOptions cr_ay_max: Reference Generator/Constant Radius/Constant Radius/ay_max
      mask TypeOptions cr_ay_stop: Reference Generator/Constant Radius/Constant Radius/ay_stop
      mask TypeOptions steerRate: Reference Generator/Fishhook/Fishhook/steerRate
      mask TypeOptions pFdbk: Reference Generator/Fishhook/Fishhook/pFdbk
      mask Callback pFdbk:
      | block = gcb;
      | pFdbkChk = get_param(block,'pFdbk');
      | if strcmp(pFdbkChk,'off')
      |     autoblksenableparameters(block,{'tDwell1'},{'pZero'},[],[],'false')
      | else
      |     autoblksenableparameters(block,{'pZero'},{'tDwell1'},[],[],'false')
      | end
      mask TypeOptions tDwell1: Reference Generator/Fishhook/Fishhook/tDwell1
      mask TypeOptions tDwell2: Reference Generator/Fishhook/Fishhook/tDwell2
      mask TypeOptions tSteer3: Reference Generator/Fishhook/Fishhook/tSteer3
      mask TypeOptions pZero: Reference Generator/Fishhook/Fishhook/pZero
      mask TypeOptions cycleVar: Reference Generator/Drive Cycle/Drive Cycle Source/cycleVar
      mask TypeOptions ax:
      | Reference Generator/Braking/Straight Maneuver Reference
      | Generator/ax
      mask TypeOptions ax_dec:
      | Reference Generator/Braking/Straight Maneuver Reference
      | Generator/ax_dec
      mask TypeOptions fixhw:
      | Reference Generator/Braking/Straight Maneuver Reference
      | Generator/fixhw
      mask TypeOptions x_brake:
      | Reference Generator/Braking/Straight Maneuver Reference
      | Generator/x_brake
      mask TypeOptions t_wot2: Reference Generator/WOT/Drive Cycle Source/t_wot2
      mask TypeOptions engine3D: 3D Engine/engine3D
      mask Callback engine3D: [~]=vdynblksrefconfig(gcb,4);
      mask TypeOptions Trailer: 3D Engine/Trailer
      mask TypeOptions SceneDesc: 3D Engine/SceneDesc
      mask Callback SceneDesc: [~] = vdynblks3Dsceneconfig(gcb);
      mask TypeOptions dt3D: 3D Engine/dt3D
      mask TypeOptions defaultPos: Recommended for scene | User-specified
      mask Callback defaultPos: [~] = vdynblksmdlWSconfig(gcb,false);
      mask TypeOptions X_o: 3D Engine/X_o | Reference Generator/Constant Radius/Constant Radius/X_o | Reference Generator/Double Lane Change/Double Lane Change/X_o | Reference Generator/Increasing Steer/Increasing Steer/X_o | Reference Generator/Sine with Dwell/Sine With Dwell/X_o | Reference Generator/Swept Sine/Swept Sine/X_o
      mask TypeOptions Y_o: 3D Engine/Y_o | Reference Generator/Constant Radius/Constant Radius/Y_o | Reference Generator/Double Lane Change/Double Lane Change/Y_o | Reference Generator/Fishhook/Fishhook/Y_o | Reference Generator/Increasing Steer/Increasing Steer/Y_o | Reference Generator/Sine with Dwell/Sine With Dwell/Y_o | Reference Generator/Swept Sine/Swept Sine/Y_o
      mask TypeOptions Z_o: 3D Engine/Z_o
      mask TypeOptions phi_o: 3D Engine/phi_o | Reference Generator/Double Lane Change/Double Lane Change/psi_o
      mask TypeOptions theta_o: 3D Engine/theta_o
      mask TypeOptions psi_o: 3D Engine/psi_o | Reference Generator/Constant Radius/Constant Radius/psi_o | Reference Generator/Fishhook/Fishhook/psi_o | Reference Generator/Increasing Steer/Increasing Steer/psi_o | Reference Generator/Sine with Dwell/Sine With Dwell/psi_o | Reference Generator/Swept Sine/Swept Sine/psi_o
      mask DialogControl modTab Prompt: vdynblks:vehdynManConstantRadius:blkDlg_modTab
      mask DialogControl configGroup Prompt: vdynblks:vehdynManConstantRadius:blkDlg_configGroup
      mask DialogControl manType Prompt: Maneuver:
      mask DialogControl manOverride Prompt: Use maneuver-specific driver, initial position, and scene
      mask DialogControl t_start Prompt: Maneuver start time, t_start [s]:
      mask DialogControl xdot_r Prompt: Longitudinal velocity reference, xdot_r:
      mask DialogControl xdotUnit Prompt: Units of velocity, xdotUnit []:
      mask DialogControl ISGroup Prompt: vdynblks:vehdynManConstantRadius:blkDlg_ISGroup
      mask DialogControl omega_hw Prompt: Handwheel rate, omega_hw [deg/s]:
      mask DialogControl theta_max Prompt: Maximum handwheel angle, theta_max [deg]:
      mask DialogControl t_stop Prompt: Steering hold time after max angle reached, t_stop [s]:
      mask DialogControl ay_max Prompt: Lateral acceleration threshold, ay_max [g]:
      mask DialogControl ay_stop Prompt: Stop simulation at lateral acceleration threshold:
      mask DialogControl DLCGroup Prompt: vdynblks:vehdynManConstantRadius:blkDlg_DLCGroup
      mask DialogControl XGate Prompt: Inertial longitudinal position of gate entrance, XGate [m]:
      mask DialogControl xStart Prompt: Distance after target speed to begin reference, xStart [m]:
      mask DialogControl vehW Prompt: Vehicle width, vehW [m]:
      mask DialogControl latoff Prompt: Lateral offset, latoff [m]:
      mask DialogControl latRefbp Prompt: Lateral reference position breakpoints [m]:
      mask DialogControl latRef Prompt: Lateral reference data, latRef [m]:
      mask DialogControl SSGroup Prompt: vdynblks:vehdynManConstantRadius:blkDlg_SSGroup
      mask DialogControl t_sweep Prompt: Swept time, t_sweep [s]:
      mask DialogControl theta_hw Prompt: Steering amplitude, theta_hw [deg]:
      mask DialogControl theta_hw_final Prompt: Final frequency, theta_hw_final [Hz]:
      mask DialogControl SDGroup Prompt: vdynblks:vehdynManConstantRadius:blkDlg_SDGroup
      mask DialogControl steerF Prompt: Steer frequency, steerF [Hz]:
      mask DialogControl steerA Prompt: Steer amplitude, steerA [deg]:
      mask DialogControl tdwell Prompt: Dwell time, tdwell [s]:
      mask DialogControl CRGroup Prompt: vdynblks:vehdynManConstantRadius:blkDlg_CRGroup
      mask DialogControl FHGroup Prompt: vdynblks:vehdynManConstantRadius:blkDlg_FHGroup
      mask DialogControl steerRate Prompt: Steer and countersteer speed, steerRate [deg/s]:
      mask DialogControl steerAFH Prompt: Steer amplitude, steerAFH, [deg]:
      mask DialogControl pFdbk Prompt: Use roll rate to determine initial steer dwell time
      mask DialogControl tDwell1 Prompt: Initial dwell time, tDwell1 [s]:
      mask DialogControl tDwell2 Prompt: Countersteer dwell time, tDwell2 [s]:
      mask DialogControl tSteer3 Prompt: Return to center time, tSteer3 [s]:
      mask DialogControl pZero Prompt: Roll rate countersteer initiation zero crossing threshold, pZero [deg/s]:
      mask DialogControl pZero Tooltip: vdynblks:vehdynManFishook:blkDlg_pZeroToolTip
      mask DialogControl DCGroup Prompt: Drive Cycle
      mask DialogControl cycleVar Prompt: Drive cycle source:
      mask DialogControl openDCbutton Prompt: Click for all configuration options
      mask DialogControl openDCbutton Callback: open_system([gcb '/Reference Generator/Drive Cycle/Drive Cycle Source'])
      mask DialogControl BGroup Prompt: Braking
      mask DialogControl ax Prompt: Longitudinal acceleration at t_start, ax [g]:
      mask DialogControl ax_dec Prompt: Longitudinal deceleration at t_brake, ax_dec [g]:
      mask DialogControl fixhw Prompt: Set handwheel angle to 0 deg after braking
      mask DialogControl x_brake Prompt: Longitudinal displacement of vehicle CG, x_brake [m]:
      mask DialogControl WOTGroup Prompt: Wide Open Throttle (WOT)
      mask DialogControl t_wot2 Prompt: Time to start deceleration, t_wot2 [s]:
      mask DialogControl simTime Prompt: Simulation time, simTime [s]:
      mask DialogControl simUpdate Prompt: vdynblks:vehdynManConstantRadius:blkDlg_simUpdate
      mask DialogControl simUpdate Callback: [~]=vdynblksrefconfig(gcb,2);
      mask DialogControl sim3DTab Prompt: vdynblks:vehdynManConstantRadius:blkDlg_sim3DTab
      mask DialogControl sim3DGroup Prompt: vdynblks:vehdynManConstantRadius:blkDlg_sim3DGroup
      mask DialogControl engine3D Prompt: 3D Engine:
      mask DialogControl SceneDesc Prompt: Scene:
      mask DialogControl dt3D Prompt: 3D Engine frame rate, dt3D [s]:
      mask DialogControl posSetupDesc Prompt: To use these initial vehicle positions, first Apply the initial values and then click Update the model workspaces with the initial values.
      mask DialogControl Z_o Prompt: Initial vertical position, Z_o [m]:
      mask DialogControl phi_o Prompt: Initial roll angle, phi_o [rad]:
      mask DialogControl theta_o Prompt: Initial pitch angle, theta_o [rad]:
      mask Display: image('vdbslibscen.png');
  Ref : Outport
  Vis : Outport  Port=2
  Fdbk : Outport  Port=3

== system VirtualVehicleTemplate/Scenarios/Reference Routing ==
  ExtDrvRef : Inport  OutDataTypeStr=Bus: VVCDrvRefBUS
  ExtDrvCmds : Inport  Port=2  OutDataTypeStr=Bus: VVCDrvCmdBUS
  ScenBus : Inport  Port=3
  Bus Assignment : BusAssignment  AssignedSignals=LngRef,LtrRef,XRef,YRef,PhiRef,CurvRef
  Bus Assignment1 : BusAssignment  AssignedSignals=SteerCmd.EnblSteerCmd,SteerCmd.SteerCmd,SteerCmd.SteerHld,SteerCmd.SteerZero,AccelCmd.EnblAccelCmd,AccelCmd.AccelCmd,AccelCmd.AccelHld,AccelCmd.AccelZero,DecelCmd.EnblDecelCmd,DecelCmd.DecelCmd,DecelCmd.DecelHld,DecelCmd.DecelZero
  Bus Creator : BusCreator  Inputs=2
  Bus Selector : BusSelector  OutputSignals=LngRef,LtrlRef,PoseRef,CurvRef
  Bus Selector1 : BusSelector  OutputSignals=EnblSteerCmd,SteerOvrCmd,SteerHld,SteerZero,EnblAccelOvr,AccelOvrCmd,AccelHld,AccelZero,EnblDecelCmd,DecelOvrCmd,DecelHld,DecelZero
  Demux : Demux  Outputs=3
  ExtDrvCmdsSwitch : Constant  Value=ExtDrvCmdsSwitch
  ExtDrvRefSwitch : Constant  Value=ExtDrvRefSwitch
  Switch : Switch  Criteria=u2 > Threshold  SaturateOnIntegerOverflow=off  InputSameDT=off
  Switch1 : Switch  Criteria=u2 > Threshold  SaturateOnIntegerOverflow=off  InputSameDT=off
  Unit Conversion1 : UnitConversion
  Unit Conversion2 : UnitConversion
  VehRef : Outport
  wires:
  Bus Selector1/9 -> Bus Assignment1/10  "<EnblDecelCmd>"
  Bus Selector/3 -> Demux/1  "<PoseRef>"
  Bus Selector/1 -> Unit Conversion2/1  "<LngRef>"
  Bus Selector1/8 -> Bus Assignment1/9  "<AccelZero>"
  Demux/2 -> Bus Assignment/5
  Bus Selector1/4 -> Bus Assignment1/5  "<SteerZero>"
  Bus Selector1/3 -> Bus Assignment1/4  "<SteerHld>"
  Bus Selector1/10 -> Bus Assignment1/11  "<DecelOvrCmd>"
  ExtDrvRef/1 -> Bus Assignment/1, Switch/1
  Bus Selector1/1 -> Bus Assignment1/2  "<EnblSteerCmd>"
  Bus Assignment/1 -> Switch/3
  Demux/1 -> Bus Assignment/4
  Demux/3 -> Bus Assignment/6
  Bus Assignment1/1 -> Switch1/3
  Bus Selector/2 -> Bus Assignment/3  "<LtrlRef>"
  Bus Selector1/7 -> Bus Assignment1/8  "<AccelHld>"
  ScenBus/1 -> Bus Selector1/1, Bus Selector/1
  Switch1/1 -> Bus Creator/2  "DrvCmd"
  Bus Selector1/12 -> Bus Assignment1/13  "<DecelZero>"
  Bus Selector1/11 -> Bus Assignment1/12  "<DecelHld>"
  Bus Selector1/2 -> Unit Conversion1/1  "<SteerOvrCmd>"
  Bus Selector1/6 -> Bus Assignment1/7  "<AccelOvrCmd>"
  ExtDrvCmds/1 -> Bus Assignment1/1, Switch1/1
  ExtDrvRefSwitch/1 -> Switch/2
  ExtDrvCmdsSwitch/1 -> Switch1/2
  Switch/1 -> Bus Creator/1  "DrvRef"
  Bus Selector/4 -> Bus Assignment/7  "<CurvRef>"
  Bus Selector1/5 -> Bus Assignment1/6  "<EnblAccelOvr>"
  Bus Creator/1 -> VehRef/1  "VehRef"
  Unit Conversion1/1 -> Bus Assignment1/3
  Unit Conversion2/1 -> Bus Assignment/2

== system VirtualVehicleTemplate/Visualization/Coordinate Systems ==
  VehFdbkIn : Inport
  ISO 8855 (Z-up) : Subsystem  VariantControl=Choice
  SAE J670 (Z-down) : Subsystem  VariantControl=ISO 8855 (Z-up)1
  VehFdbk : Outport

== system VirtualVehicleTemplate/Visualization/DataLogging ==
  VehFdbk : Inport
  Bus Selector : BusSelector  OutputSignals=Driver.SteerFdbk
  Terminator : Terminator
  wires:
  VehFdbk/1 -> Bus Selector/1
  Bus Selector/1 -> Terminator/1  "<SteerFdbk>"

== system VirtualVehicleTemplate/Visualization/Emission Calculations ==
  VehSpd : Inport
  TP HC Mass Flow : Inport  Port=2
  TP CO Mass Flow : Inport  Port=3
  TP NOx Mass Flow : Inport  Port=4
  TP CO2 Mass Flow : Inport  Port=5
  Integrator{,1..4} (5 alike) : Integrator
  Kg to g : Gain  Gain=1000
  "Kg to g " : Gain  Gain=1000
  "Kg to g  " : Gain  Gain=1000
  "Kg to g   " : Gain  Gain=1000
  L/100 Km Calc{,1..3} (4 alike) : Product  Inputs=/*
  Rate Transition{,1..3} (4 alike) : RateTransition  Deterministic=off
  Saturation : Saturate  UpperLimit=Inf  LowerLimit=0.2  ZeroCross=off
  Saturation1 : Saturate  UpperLimit=Inf  LowerLimit=1  ZeroCross=off
  Signal Specification5 : SignalSpecification  Unit=m/s
  Unit Conversion5 : UnitConversion
  m to km : Gain  Gain=0.001
  m to mi : Gain  Gain=0.000621371
  TP HC Mass : Outport  VectorParamsAs1DForOutWhenUnconnected=off
  TP CO Mass : Outport  Port=2  VectorParamsAs1DForOutWhenUnconnected=off
  TP NOx Mass : Outport  Port=3  VectorParamsAs1DForOutWhenUnconnected=off
  TP CO2 Mass : Outport  Port=4  VectorParamsAs1DForOutWhenUnconnected=off
  wires:
  L/100 Km Calc/1 -> Rate Transition/1
  m to mi/1 -> Saturation/1
  Saturation/1 -> L/100 Km Calc2/1, L/100 Km Calc1/1, L/100 Km Calc/1
  TP HC Mass Flow/1 -> Integrator1/1
  Integrator1/1 -> Kg to g/1
  Integrator/1 -> m to km/1, m to mi/1
  Kg to g/1 -> L/100 Km Calc/2
  TP CO Mass Flow/1 -> Integrator2/1
  Integrator2/1 -> "Kg to g "/1
  "Kg to g "/1 -> L/100 Km Calc1/2
  TP NOx Mass Flow/1 -> Integrator3/1
  Integrator3/1 -> "Kg to g  "/1
  "Kg to g  "/1 -> L/100 Km Calc2/2
  L/100 Km Calc1/1 -> Rate Transition1/1
  L/100 Km Calc2/1 -> Rate Transition2/1
  TP CO2 Mass Flow/1 -> Integrator4/1
  Integrator4/1 -> "Kg to g   "/1
  "Kg to g   "/1 -> L/100 Km Calc3/2
  L/100 Km Calc3/1 -> Rate Transition3/1
  Saturation1/1 -> L/100 Km Calc3/1
  m to km/1 -> Saturation1/1
  Rate Transition/1 -> TP HC Mass/1  "TP HC Mass (g/mi)"
  Rate Transition1/1 -> TP CO Mass/1  "TP CO Mass (g/mi)"
  Rate Transition2/1 -> TP NOx Mass/1  "TP NOx Mass (g/mi)"
  Rate Transition3/1 -> TP CO2 Mass/1  "TP CO2 Mass (g/km)"
  Unit Conversion5/1 -> Signal Specification5/1
  VehSpd/1 -> Unit Conversion5/1
  Signal Specification5/1 -> Integrator/1
